simulink model "openWaterModel"  (R2020a)
settings: Solver=FixedStepAuto  StartTime=0.0  StopTime=inf  FixedStep=Ts  RelTol=1e-3  EnableMultiTasking=on
values from neighbouring files (symbols this model uses):
  ctrlMap =     [init_Kite.mat]
  Ts = 0.01    [init_Kite.mat]
undefined symbols (not defined in the file or in its folder): initializeBussesFromBlock, IO397, standard
libraries: xpcutilitieslib x172, hdlsllib x100, simulink x36, dspsigops x13, slrtlib x4, xpcseriallib x3, speedgoatlib_fpga_analog_io x2, xpcrtudplib x2, speedgoatlib_fpga_dio x1, speedgoatlib_fpga_quadrature x1, speedgoatlib_IO581 x1, speedgoatlib_fpga x1
(part 2 of 4)

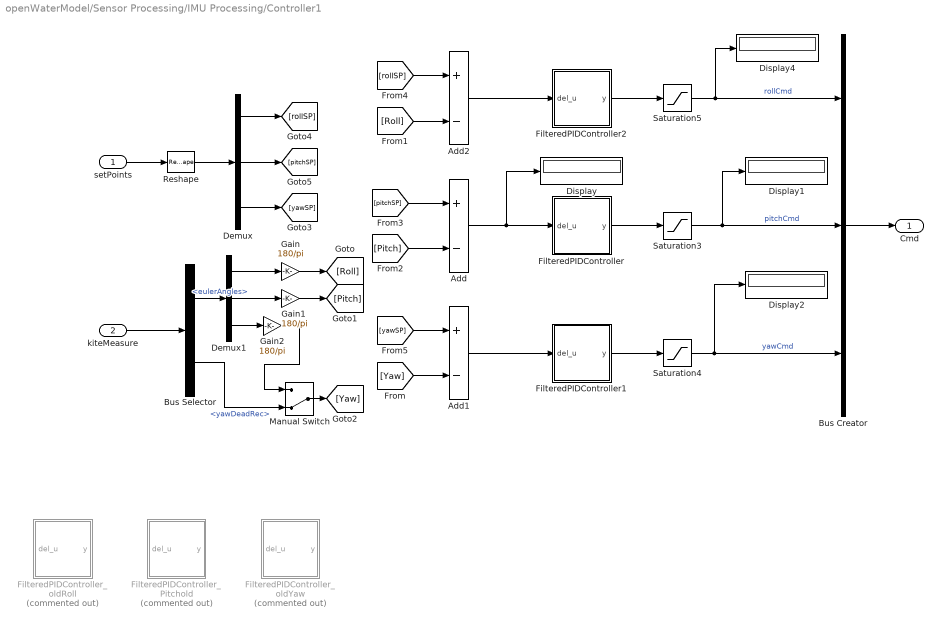
== system openWaterModel/Sensor Processing/IMU Processing/Controller1 ==
  setPoints : Inport
  kiteMeasure : Inport  Port=2
  Add : Sum  Inputs=+-
  Add1 : Sum  Inputs=+-
  Add2 : Sum  Inputs=+-
  Bus Creator : BusCreator  Inputs=3
  Bus Selector : BusSelector  OutputSignals=eulerAngles,yawDeadRec
  Demux : Demux  Outputs=3
  Demux1 : Demux  Outputs=3
  Display{,1..2,4} (4 alike) : Display
  FilteredPIDController : Subsystem  mask{Kp=1, Kd=0, tau=1, Ki=0}
      mask prompts: Kp "Proportional Gain"; Kd "Derivative Gain"; tau "Time constant"; Ki "Integral Gain"
  FilteredPIDController1 : Subsystem  mask{Kp=1, Kd=0, tau=1, Ki=0}
      mask prompts: Kp "Proportional Gain"; Kd "Derivative Gain"; tau "Time constant"; Ki "Integral Gain"
  FilteredPIDController2 : Subsystem  mask{Kp=1, Kd=0, tau=1, Ki=0}
      mask prompts: Kp "Proportional Gain"; Kd "Derivative Gain"; tau "Time constant"; Ki "Integral Gain"
  FilteredPIDController_Pitchold : Subsystem  Commented=on  mask{Kp=1, Kd=0, tau=1, Ki=0}
      mask prompts: Kp "Proportional Gain"; Kd "Derivative Gain"; tau "Time constant"; Ki "Integral Gain"
  FilteredPIDController_oldRoll : Subsystem  Commented=on  mask{Kp=1, Kd=0, tau=1, Ki=0}
      mask prompts: Kp "Proportional Gain"; Kd "Derivative Gain"; tau "Time constant"; Ki "Integral Gain"
  FilteredPIDController_oldYaw : Subsystem  Commented=on  mask{Kp=1, Kd=0, tau=1, Ki=0}
      mask prompts: Kp "Proportional Gain"; Kd "Derivative Gain"; tau "Time constant"; Ki "Integral Gain"
  Gain : Gain  Gain=180/pi
  Gain1 : Gain  Gain=180/pi
  Gain2 : Gain  Gain=180/pi
  Manual Switch : ManualSwitch  CurrentSetting=0
  Reshape : Reshape  OutputDimensionality=Column vector (2-D)
  Saturation3 : Saturate  UpperLimit=30  LowerLimit=-30
  Saturation4 : Saturate  UpperLimit=29  LowerLimit=-29
  Saturation5 : Saturate  UpperLimit=30  LowerLimit=-30
  Cmd : Outport
  wires:
  [Pitch] -> Add/2
  [Yaw] -> Add1/2
  [yawSP] -> Add1/1
  Demux/3 -> [yawSP]
  [pitchSP] -> Add/1
  kiteMeasure/1 -> Bus Selector/1
  Saturation4/1 -> Display2/1, Bus Creator/3  "yawCmd"
  Saturation5/1 -> Display4/1, Bus Creator/1  "rollCmd"
  Bus Creator/1 -> Cmd/1
  Reshape/1 -> Demux/1
  setPoints/1 -> Reshape/1
  Add/1 -> FilteredPIDController/1(del_u), Display/1
  [rollSP] -> Add2/1
  [Roll] -> Add2/2
  Demux/2 -> [pitchSP]
  Demux/1 -> [rollSP]
  Bus Selector/1 -> Demux1/1  "<eulerAngles>"
  Demux1/1 -> Gain/1
  Demux1/2 -> Gain1/1
  Demux1/3 -> Gain2/1
  Saturation3/1 -> Display1/1, Bus Creator/2  "pitchCmd"
  FilteredPIDController/1(y) -> Saturation3/1
  FilteredPIDController2/1(y) -> Saturation5/1
  Add2/1 -> FilteredPIDController2/1(del_u)
  FilteredPIDController1/1(y) -> Saturation4/1
  Add1/1 -> FilteredPIDController1/1(del_u)
  Gain/1 -> [Roll]
  Gain1/1 -> [Pitch]
  Bus Selector/2 -> Manual Switch/2  "<yawDeadRec>"
  Gain2/1 -> Manual Switch/1
  Manual Switch/1 -> [Yaw]

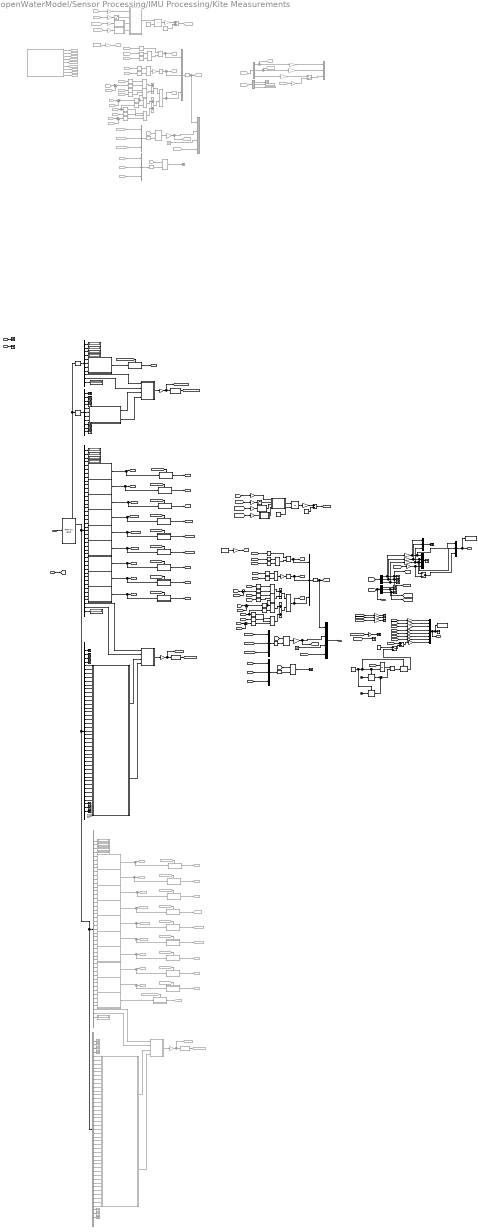
== system openWaterModel/Sensor Processing/IMU Processing/Kite Measurements  ==
  note: Dead Reconing Yaw
  note: Tranformation from IMU euler angles w.r.t NED to Body euler angles w.r.t Ground. Transformation from acc / angular rate in the IMU to acc / angular rate in the Body.
  note: Debug
  note: Tranformation from IMU euler angles w.r.t NED to Body euler angles w.r.t Ground. Transformation from acc / angular rate in the IMU to acc / angular rate in the Body.
  note: Serial Data Recieve
  serialData : Inport
  DcM : Inport  Port=2
  gndStnEul : Inport  Port=3
  winchCmd : Inport  Port=4
  Add : Sum  Commented=on
  Add1 : Sum  Commented=on
  Add2 : Sum  Commented=on  Inputs=+-
  Add3 : Sum
  Add4 : Sum
  Add5 : Sum  Inputs=+-
  Add6 : Sum  Inputs=+-
  Bus Creator1 : BusCreator  Commented=on  Inputs=4
  Bus Creator2 : BusCreator  Inputs=4
  Cast To Boolean : DataTypeConversion  OutDataTypeStr=boolean
  Cast To Boolean1 : DataTypeConversion  OutDataTypeStr=boolean
  Cast To Boolean2 : DataTypeConversion  Commented=on  OutDataTypeStr=boolean
  Clock : Clock
  Clock1 : Clock
  Constant : Constant  Value=0
  Cos{1..2,4,6,10..11} (6 alike) : Trigonometry  Commented=on
  Cos{3,5,7..9,12..13} (7 alike) : Trigonometry  Commented=on  Operator=cos
  Cos{14..16,19,21,23} (6 alike) : Trigonometry
  Cos{17..18,20,22,24..26} (7 alike) : Trigonometry  Operator=cos
  Demux : Demux  Outputs=43
  Demux1 : Demux  Commented=on  Outputs=3
  Demux2 : Demux  Commented=on  Outputs=3
  Demux3 : Demux  Outputs=3
  Demux4 : Demux  Outputs=3
  Demux5 : Demux  Outputs=43
  Demux6 : Demux  Outputs=11
  Demux7 : Demux  Outputs=11
  Demux8 : Demux  Commented=on  Outputs=47
  Demux9 : Demux  Commented=on  Outputs=47
  Display{,1..9} (10 alike) : Display
      Display settings: Format=hex (Stored Integer)
      Display2 settings: Format=hex (Stored Integer)
      Display3 settings: Format=hex (Stored Integer)
      Display4 settings: Format=hex (Stored Integer)
      Display5 settings: Format=hex (Stored Integer)
      Display6 settings: Format=hex (Stored Integer)
      Display7 settings: Format=hex (Stored Integer)
      Display8 settings: Format=hex (Stored Integer)
  Display{10..14} (5 alike) : Display  Commented=on
      Display10 settings: Format=hex (Stored Integer)
      Display12 settings: Format=hex (Stored Integer)
      Display13 settings: Format=hex (Stored Integer)
      Display14 settings: Format=hex (Stored Integer)
  Divide : Product  Inputs=*/
  Enabled Subsystem : Subsystem  TreatAsAtomicUnit=on
  Enabled Subsystem1 : Subsystem  TreatAsAtomicUnit=on
  Enabled Subsystem10 : Subsystem  Commented=on  TreatAsAtomicUnit=on
  Enabled Subsystem11 : Subsystem  Commented=on  TreatAsAtomicUnit=on
  Enabled Subsystem12 : Subsystem  Commented=on  TreatAsAtomicUnit=on
  Enabled Subsystem13 : Subsystem  Commented=on  TreatAsAtomicUnit=on
  Enabled Subsystem14 : Subsystem  Commented=on  TreatAsAtomicUnit=on
  Enabled Subsystem15 : Subsystem  Commented=on  TreatAsAtomicUnit=on
  Enabled Subsystem16 : Subsystem  Commented=on  TreatAsAtomicUnit=on
  Enabled Subsystem17 : Subsystem  Commented=on  TreatAsAtomicUnit=on
  Enabled Subsystem18 : Subsystem  Commented=on  TreatAsAtomicUnit=on
  Enabled Subsystem19 : Subsystem  Commented=on  TreatAsAtomicUnit=on
  Enabled Subsystem2 : Subsystem  TreatAsAtomicUnit=on
  Enabled Subsystem3 : Subsystem  TreatAsAtomicUnit=on
  Enabled Subsystem4 : Subsystem  TreatAsAtomicUnit=on
  Enabled Subsystem5 : Subsystem  TreatAsAtomicUnit=on
  Enabled Subsystem6 : Subsystem  TreatAsAtomicUnit=on
  Enabled Subsystem7 : Subsystem  TreatAsAtomicUnit=on
  Enabled Subsystem8 : Subsystem  TreatAsAtomicUnit=on
  Enabled Subsystem9 : Subsystem  TreatAsAtomicUnit=on
  "FIFO bin read " : xpcseriallib/FIFO bin read   header={[0x47 0xBB 0x3C 0x2B] [0x58 0xCC 0x4D 0x3C]}  lengths=[42 10]  hold=Hold last output if no new data  enable=off  maxsize=42  outputtype=8 bit uint null terminated  sampletime=0.01
      settings: SourceProductBaseCode=XP
  Fletcher16 Checksum : Subsystem
  Fletcher16 Checksum1 : Subsystem
  Fletcher16 Checksum2 : Subsystem  Commented=on
  From1 : From  Commented=on  GotoTag=yawDeadRec
  From10 : From  Commented=on  GotoTag=DcM
  From2 : From  Commented=on  GotoTag=eulVector
  From3 : From  Commented=on  GotoTag=rateVector
  From35 : From  Commented=on  GotoTag=psiG
  From{36,40,42..43,53} (5 alike) : From  Commented=on  GotoTag=thetaIMU
  From37 : From  Commented=on  GotoTag=DcM
  From38 : From  Commented=on  GotoTag=pIMU
  From{39,41,44,54..55} (5 alike) : From  Commented=on  GotoTag=phiIMU
  From4 : From  Commented=on  GotoTag=roll
  From{45,59..60,72,87,89..91,97} (9 alike) : From  Commented=on  GotoTag=checksumEnable
  From46 : From  Commented=on  GotoTag=rIMU
  From47 : From  Commented=on  GotoTag=axIMU
  From48 : From  Commented=on  GotoTag=ayIMU
  From49 : From  Commented=on  GotoTag=azIMU
  From5 : From  Commented=on  GotoTag=pitch
  From50 : From  Commented=on  GotoTag=psiG
  From51 : From  Commented=on  GotoTag=psiIMU
  From52 : From  Commented=on  GotoTag=psiIMU
  From56 : From  Commented=on  GotoTag=psiG
  From57 : From  Commented=on  GotoTag=psiIMU
  From58 : From  Commented=on  GotoTag=qIMU
  From6 : From  Commented=on  GotoTag=q
  From7 : From  Commented=on  GotoTag=r
  From8 : From  Commented=on  GotoTag=yawDeadRec
  From92 : From  Commented=on  GotoTag=checksumEnablePressure
  Gain : Gain  Commented=on  Gain=-1
  Gain1 : Gain  Gain=-1
  Gain{10,15,21..23} (5 alike) : Gain  Commented=on  Gain=180/pi
  Gain{4,11..14,25..27,32..33} (10 alike) : Gain  Gain=180/pi
  Gain16 : Gain  Commented=on
  Gain{3,5,17..19,24,29..30} (8 alike) : Gain
  Gain2 : Gain  Commented=on  Gain=-1
  Gain20 : Gain  Gain=-1
  Gain28 : Gain  Gain=1.01972
  Gain31 : Gain  Commented=on
  Gain{34..37} (4 alike) : Gain  Gain=pi/180
  Gain{6..9} (4 alike) : Gain  Commented=on  Gain=pi/180
  Goto18 : Goto  Commented=on  GotoTag=phiIMU
  Goto19 : Goto  Commented=on  GotoTag=psiIMU
  Goto20 : Goto  Commented=on  GotoTag=pIMU
  Goto22 : Goto  Commented=on  GotoTag=qIMU
  Goto23 : Goto  Commented=on  GotoTag=rIMU
  Goto24 : Goto  Commented=on  GotoTag=axIMU
  Goto25 : Goto  Commented=on  GotoTag=ayIMU
  Goto26 : Goto  Commented=on  GotoTag=azIMU
  Goto27 : Goto  Commented=on  GotoTag=thetaIMU
  Goto28 : Goto  Commented=on  GotoTag=psiG
  Goto29 : Goto  Commented=on  GotoTag=phi
  Goto3 : Goto  Commented=on  GotoTag=roll
  Goto30 : Goto  Commented=on  GotoTag=theta
  Goto31 : Goto  Commented=on  GotoTag=psi
  Goto32 : Goto  Commented=on  GotoTag=eulVector
  Goto33 : Goto  Commented=on  GotoTag=rateVector
  Goto4 : Goto  Commented=on  GotoTag=pitch
  Goto49 : Goto  Commented=on  GotoTag=thetaRaw
  Goto5 : Goto  Commented=on  GotoTag=q
  Goto50 : Goto  Commented=on  GotoTag=psiRaw
  Goto51 : Goto  Commented=on  GotoTag=pRaw
  Goto52 : Goto  Commented=on  GotoTag=qRaw
  Goto53 : Goto  Commented=on  GotoTag=rRaw
  Goto55 : Goto  Commented=on  GotoTag=ayRaw
  Goto56 : Goto  Commented=on  GotoTag=azRaw
  Goto57 : Goto  Commented=on  GotoTag=checksumEnable
  Goto58 : Goto  Commented=on  GotoTag=phiIMU
  Goto59 : Goto  Commented=on  GotoTag=psiIMU
  Goto6 : Goto  Commented=on  GotoTag=r
  Goto60 : Goto  Commented=on  GotoTag=pIMU
  Goto61 : Goto  Commented=on  GotoTag=CSisMatch
  Goto62 : Goto  Commented=on  GotoTag=qIMU
  Goto63 : Goto  Commented=on  GotoTag=rIMU
  Goto64 : Goto  Commented=on  GotoTag=axIMU
  Goto66 : Goto  Commented=on  GotoTag=ayIMU
  Goto67 : Goto  Commented=on  GotoTag=azIMU
  Goto68 : Goto  Commented=on  GotoTag=thetaIMU
  Goto69 : Goto  Commented=on  GotoTag=axRaw
  Goto7 : Goto  Commented=on  GotoTag=yawDeadRec
  Goto70 : Goto  Commented=on  GotoTag=phiRaw
  Goto71 : Goto  Commented=on  GotoTag=pres
  Ground : Ground  Commented=on
  Ground1 : Ground
  Ground2 : Ground  Commented=on
  Integrator : Integrator  Commented=on  ExternalReset=either
  Integrator1 : Integrator  ExternalReset=either
  Integrator2 : Integrator  ExternalReset=either
  MATLAB Function : MATLAB Function  Commented=on  TreatAsAtomicUnit=on
  MATLAB Function1 : MATLAB Function  Commented=on  TreatAsAtomicUnit=on
  MATLAB Function2 : MATLAB Function  Commented=on  TreatAsAtomicUnit=on
  MATLAB Function3 : MATLAB Function  TreatAsAtomicUnit=on
  MATLAB Function4 : MATLAB Function  TreatAsAtomicUnit=on
  MATLAB Function5 : MATLAB Function  TreatAsAtomicUnit=on
  MATLAB Function6 : MATLAB Function  TreatAsAtomicUnit=on
  MATLAB Function7 : MATLAB Function  TreatAsAtomicUnit=on
  MATLAB Function8 : MATLAB Function  Commented=on  TreatAsAtomicUnit=on
  Manual Switch : ManualSwitch  Commented=on  CurrentSetting=0
  Manual Switch1 : ManualSwitch  CurrentSetting=0
  Manual Switch2 : ManualSwitch
  Matrix Multiply1 : Product  Multiplication=Matrix(*)
  Matrix Multiply2 : Product  Commented=on  Multiplication=Matrix(*)
  Matrix Multiply3 : Product  Commented=on  Multiplication=Matrix(*)
  Matrix Multiply4 : Product  Multiplication=Matrix(*)
  Mux{,5..7} (4 alike) : Mux  Commented=on  Inputs=3
  Mux{1,4,8..10} (5 alike) : Mux  Inputs=3
  Mux2 : Mux
  Mux3 : Mux  Inputs=8
  PoolToNorthAngle : Constant  Commented=on  Value=2.4070
  PoolToNorthAngle1 : Constant  Value=2.4070
  Product{1..2,5..6} (4 alike) : Product  Commented=on
  Product10 : Product  Inputs=3
  Product{7..8,11..12} (4 alike) : Product
  Product3 : Product  Commented=on  Inputs=3
  Product4 : Product  Commented=on  Inputs=3
  Product9 : Product  Inputs=3
  Reshape1 : Reshape  OutputDimensionality=Column vector (2-D)
  Reshape2 : Reshape  Commented=on  OutputDimensionality=Column vector (2-D)
  Reshape3 : Reshape  Commented=on  OutputDimensionality=Column vector (2-D)
  Reshape4 : Reshape  Commented=on  OutputDimensionality=Column vector (2-D)
  Reshape5 : Reshape  OutputDimensionality=Column vector (2-D)
  Reshape6 : Reshape  OutputDimensionality=Column vector (2-D)
  Sample and Hold : dspsigops/Sample and Hold  trig=Rising edge  initCond=0  latchinput=off
  Sample and Hold1 : dspsigops/Sample and Hold  trig=Falling edge  initCond=999999  latchinput=off
  Sample and Hold2 : dspsigops/Sample and Hold  trig=Falling edge  initCond=0  latchinput=off
  Saturation : Saturate  Commented=on  UpperLimit=pi/2-0.1  LowerLimit=-pi/2+0.1
  Saturation1 : Saturate  UpperLimit=pi/2-0.1  LowerLimit=-pi/2+0.1
  Scope 1 : slrtlib/Displays and Logging/Scope   scopeno=3  scopetype=Target  autostart=on  viewmode=Numerical  formatstr='%15.6f'  grid=on  ylimits=[-100,100]  nosamples=scopeSamples  noprepostsamples=0  interleave=scopeDecimaton  triggermode=FreeRun  triggersignal=1  trigsignalfromport=off  triggerlevel=0.0  triggerslope=Either  triggerscope=1  triggersample=0  filename=data.dat  mode=Lazy  writesize=512  autorestart=off  dynamicfilemode=off  maxwritefilesize=512*1024^2
  Scope 2 : slrtlib/Displays and Logging/Scope   scopeno=1  scopetype=Target  autostart=on  viewmode=Graphical sliding  formatstr='%15.6f'  grid=on  ylimits=[-100,100]  nosamples=scopeSamples  noprepostsamples=0  interleave=scopeDecimaton  triggermode=FreeRun  triggersignal=1  trigsignalfromport=off  triggerlevel=0.0  triggerslope=Either  triggerscope=1  triggersample=0  filename=data.dat  mode=Lazy  writesize=512  autorestart=off  dynamicfilemode=off  maxwritefilesize=512*1024^2
  Selector : Selector  InputPortWidth=43  IndexOptions=Index vector (dialog)  Indices=[1 2 3 4 5 6 7 8 9 10 11]  OutputSizes=1
  Selector1 : Selector  InputPortWidth=43  IndexOptions=Index vector (dialog)  Indices=[1 2 3 4 5 6 7 8 9 10 11]  OutputSizes=1
  Serial Data Recieve : Subsystem  Commented=on
  Sin1 : Trigonometry
  Sin4 : Trigonometry  Commented=on
  Sum : Sum  Inputs=|-+
  Sum1 : Sum  Commented=on  Inputs=|+-
  Sum2 : Sum  Commented=on  Inputs=|+-
  Sum3 : Sum  Commented=on  Inputs=|+-
  Sum4 : Sum  Inputs=|+-
  Sum5 : Sum  Inputs=|+-
  Sum6 : Sum  Inputs=|+-
  Terminator{,1..3,5..6,8..22,27..29,33..39} (31 alike) : Terminator
  Terminator{4,7,23..26,30..32} (9 alike) : Terminator  Commented=on
  Trigonometric Function : Trigonometry  Commented=on  Operator=atan2
  Trigonometric Function1 : Trigonometry  Commented=on  Operator=asin
  Trigonometric Function2 : Trigonometry  Commented=on  Operator=atan2
  Trigonometric Function3 : Trigonometry  Operator=atan2
  Trigonometric Function4 : Trigonometry  Operator=asin
  Trigonometric Function5 : Trigonometry  Operator=atan2
  airPressure : Constant  Value=1022
  binary2double : Subsystem
  binary2double1 : Subsystem
  binary2double10 : Subsystem  Commented=on
  binary2double11 : Subsystem  Commented=on
  binary2double12 : Subsystem  Commented=on
  binary2double13 : Subsystem  Commented=on
  binary2double14 : Subsystem  Commented=on
  binary2double15 : Subsystem  Commented=on
  binary2double16 : Subsystem  Commented=on
  binary2double17 : Subsystem  Commented=on
  binary2double18 : Subsystem  Commented=on
  binary2double19 : Subsystem  Commented=on
  binary2double2 : Subsystem
  binary2double3 : Subsystem
  binary2double4 : Subsystem
  binary2double5 : Subsystem
  binary2double6 : Subsystem
  binary2double7 : Subsystem
  binary2double8 : Subsystem
  binary2double9 : Subsystem
  eulRates : Gain  Gain=180/pi
  yawBias : Constant  Commented=on  Value=0
  yawBias1 : Constant  Value=0
  yawEstimateTrigger : Constant  Commented=on  Value=0
  yawEstimateTrigger1 : Constant
  kiteMeasure : Outport
  eul : Outport  Port=2
  angVel : Outport  Port=3
  MC_rawData : Outport  Port=4
  wires:
  From2/1 -> Demux1/1
  From3/1 -> Demux2/1
  Demux1/3 -> Gain23/1
  Demux1/1 -> Gain21/1, Goto3/1
  Demux2/3 -> Goto6/1  "r"
  Demux2/2 -> Goto5/1  "q"
  Demux2/1 -> Terminator4/1  "p"
  Gain9/1 -> MATLAB Function1/1(u)  "kiteYawRate_rad"
  Gain8/1 -> MATLAB Function2/1(u)  "kitePitchRate_rad"
  From6/1 -> Gain8/1
  From5/1 -> Gain7/1
  Saturation/1 -> MATLAB Function/2(theta)  "kitePitch_rad"
  Gain6/1 -> MATLAB Function/1(phi)  "kiteRoll_rad"
  Integrator/1 -> Gain10/1
  From7/1 -> Gain9/1
  From4/1 -> Gain6/1
  Gain7/1 -> Saturation/1
  yawEstimateTrigger/1 -> Integrator/2
  MATLAB Function/1(psi_dot) -> Integrator/1
  yawBias/1 -> Add/2
  Add/1 -> Goto7/1
  Gain10/1 -> Add/1  "rollRaw"
  MATLAB Function1/1(y) -> MATLAB Function/4(r)
  MATLAB Function2/1(y) -> MATLAB Function/3(q)
  Gain21/1 -> Mux/1  "rollDeg"
  Gain22/1 -> Mux/2  "pitchDeg"
  Gain23/1 -> Manual Switch/1  "yawIMU"
  Gain16/1 -> Manual Switch/2  "yawDeadRec"
  PoolToNorthAngle/1 -> Gain2/1
  Trigonometric Function/1 -> Mux5/1, Goto29/1
  Product2/1 -> Gain/1
  Cos2/1 -> Product2/1
  Cos3/1 -> Product2/2
  From42/1 -> Cos3/1
  From41/1 -> Cos2/1
  Trigonometric Function1/1 -> Mux5/2, Goto30/1
  Add2/1 -> Trigonometric Function2/1
  Sin4/1 -> Product4/1
  From44/1 -> Cos7/1, Sin4/1
  Mux5/1 -> Reshape2/1
  Trigonometric Function2/1 -> Goto31/1, Mux5/3
  Gain15/1 -> Goto33/1, Bus Creator1/2  "gyroRates"
  From58/1 -> Mux6/2
  Ground2/1 -> Bus Creator1/3  "Pressure (Pa)"
  From37/1 -> Matrix Multiply2/1
  Reshape3/1 -> Matrix Multiply2/2
  Reshape2/1 -> Bus Creator1/1, Goto32/1  "eulerAngles"
  Mux6/1 -> Reshape3/1
  Matrix Multiply2/1 -> Gain15/1
  From46/1 -> Mux6/3
  From38/1 -> Mux6/1
  From47/1 -> Mux7/1
  From49/1 -> Mux7/3
  Mux7/1 -> Reshape4/1
  Reshape4/1 -> Matrix Multiply3/2
  From10/1 -> Matrix Multiply3/1
  From48/1 -> Mux7/2
  Matrix Multiply3/1 -> Terminator7/1  "accBody"
  Gain/1 -> Trigonometric Function1/1
  Product1/1 -> Trigonometric Function/2
  Cos1/1 -> Trigonometric Function/1
  From36/1 -> Cos1/1
  From39/1 -> Cos8/1
  From40/1 -> Cos9/1
  Cos9/1 -> Product1/2
  Cos8/1 -> Product1/1
  From50/1 -> Sum1/1
  From51/1 -> Sum1/2
  Sum1/1 -> Cos5/1
  Cos5/1 -> Product4/3
  From43/1 -> Cos6/1
  Cos6/1 -> Product4/2
  Product4/1 -> Add1/2
  Product5/1 -> Add1/1
  Cos7/1 -> Product5/2
  Cos10/1 -> Product3/3, Product5/1
  From52/1 -> Sum2/2
  From35/1 -> Sum2/1
  Sum2/1 -> Cos10/1
  Add1/1 -> Trigonometric Function2/2
  From53/1 -> Cos4/1
  From54/1 -> Cos11/1
  Cos11/1 -> Product3/2
  Cos4/1 -> Product3/1
  Product3/1 -> Add2/2
  From55/1 -> Cos12/1
  From56/1 -> Sum3/1
  From57/1 -> Sum3/2
  Sum3/1 -> Cos13/1
  Product6/1 -> Add2/1
  Cos13/1 -> Product6/2
  Cos12/1 -> Product6/1
  Gain2/1 -> Goto28/1
  From8/1 -> Gain16/1
  From1/1 -> Bus Creator1/4  "yawDeadRec"
  Manual Switch/1 -> Mux/3  "yawDeg"
  Demux1/2 -> Goto4/1, Gain22/1
  Serial Data Recieve/1(rawRollChecked) -> Goto18/1
  Serial Data Recieve/2(rawPitchChecked) -> Goto27/1
  Serial Data Recieve/3(rawRollChecked1) -> Goto19/1
  Serial Data Recieve/4(rawPchecked) -> Goto20/1
  Serial Data Recieve/5(rawQchecked) -> Goto22/1
  Serial Data Recieve/6(rawRchecked) -> Goto23/1
  Serial Data Recieve/7(rawAxChecked) -> Goto24/1
  Serial Data Recieve/8(rawAyChecked) -> Goto25/1
  Serial Data Recieve/9(rawAzChecked) -> Goto26/1
  gndStnEul/1 -> Terminator/1
  winchCmd/1 -> Terminator1/1
  airPressure/1 -> Manual Switch2/1
  Enabled Subsystem10/1(Out1) -> Goto58/1  "rawRollChecked"
  Demux6/4 -> Display5/1
  Gain12/1 -> Terminator29/1  "p"
  Demux9/24 -> Fletcher16 Checksum2/20(In20)
  Demux4/3 -> [kiteR], Terminator36/1  "kiteR"
  Demux/7 -> binary2double/3(In3)
  Gain34/1 -> MATLAB Function3/1(phi)  "kiteRoll_rad"
  [yawDeadRec] -> Bus Creator2/4  "yawDeadRec"
  Demux8/16 -> binary2double12/4(In4)
  Demux8/37 -> binary2double18/1(In1)
  [thetaIMU] -> Cos14/1
  Demux9/13 -> Fletcher16 Checksum2/9(In9)
  Demux9/39 -> Fletcher16 Checksum2/35(In35)
  Cos23/1 -> Product10/2
  Demux8/27 -> binary2double15/3(In3)
  Demux9/42 -> Fletcher16 Checksum2/38(In38)
  Add4/1 -> Trigonometric Function5/2
  Cast To Boolean2/1 -> Goto57/1
  Demux8/4 -> Display10/1
  binary2double16/1(Double) -> Enabled Subsystem16/1(Double), Goto69/1  "rawAx"
  Demux5/25 -> Fletcher16 Checksum/21(In21)
  Mux4/1 -> Terminator38/1
  [DcM] -> Matrix Multiply1/1
  Gain31/1 -> Goto61/1, Cast To Boolean2/1  "checksumIsMatch"
  Reshape1/1 -> Bus Creator2/1, [eulVector]  "eulerAngles"
  From91/1 -> Enabled Subsystem18/Enable
  Demux5/14 -> Fletcher16 Checksum/10(In10)
  Demux/11 -> binary2double1/3(In3)
  Add6/1 -> Gain28/1
  Demux3/2 -> [kitePitch], Terminator5/1, Gain26/1  "kitePitch"
  Gain11/1 -> Mux3/1  "phi"
  Demux/41 -> MATLAB Function6/1(cSumInB1)  "cSumInB1"
  Demux/28 -> binary2double5/4(In4)
  Demux8/24 -> binary2double14/4(In4)
  Mux2/1 -> Terminator15/1
  Demux7/1 -> Terminator3/1
  Enabled Subsystem1/1(Out1) -> [thetaIMU]  "rawPitchChecked"
  [thetaIMU] -> Cos26/1
  Demux6/10 -> MATLAB Function7/2(cSumInB2)
  Gain37/1 -> MATLAB Function4/1(u)  "kiteYawRate_rad"
  [pRaw] -> Gain12/1  "pRaw"
  [checksumEnable] -> Enabled Subsystem3/Enable
  [checksumEnable] -> Enabled Subsystem6/Enable
  [ayIMU] -> Mux10/2
  binary2double3/1(Double) -> Enabled Subsystem3/1(Double), [pRaw]  "rawP"
  [checksumEnable] -> Enabled Subsystem8/Enable
  Gain24/1 -> [CSisMatch], Cast To Boolean/1  "checksumIsMatch"
  Demux8/43 -> binary2double19/3(In3)
  [rIMU] -> Mux9/3
  From59/1 -> Enabled Subsystem12/Enable
  Matrix Multiply1/1 -> eulRates/1
  Gain33/1 -> Mux3/3  "psi"
  MATLAB Function3/1(psi_dot) -> Integrator1/1
  [pres] -> Gain17/1
  Mux9/1 -> Reshape5/1
  [pIMU] -> Mux9/1
  [phiIMU] -> Cos19/1
  Trigonometric Function3/1 -> Mux8/1, [phi]
  Demux9/9 -> Fletcher16 Checksum2/5(In5)
  Demux9/11 -> Fletcher16 Checksum2/7(In7)
  [rRaw] -> Gain14/1  "rRaw"
  MATLAB Function6/1(checksumIsMatching) -> Gain24/1
  Mux8/1 -> Reshape1/1
  Demux8/5 -> binary2double10/1(In1)
  Demux8/19 -> binary2double13/3(In3)
  [ayRaw] -> Gain18/1
  Demux5/6 -> Fletcher16 Checksum/2(In2)
  Cast To Boolean/1 -> [checksumEnable]
  [psiG] -> Sum4/1
  Manual Switch1/1 -> Mux1/3  "yawChosen"
  From87/1 -> Enabled Subsystem15/Enable
  MATLAB Function4/1(y) -> MATLAB Function3/4(r)
  binary2double9/1(Double) -> Enabled Subsystem9/1(Double)  "rawPressure"
  Demux/40 -> binary2double8/4(In4)
  [checksumEnablePressure] -> Enabled Subsystem9/Enable
  [kiteRoll] -> Gain34/1
  Demux/15 -> binary2double2/3(In3)
  Cos17/1 -> Product12/1
  binary2double7/1(Double) -> Enabled Subsystem7/1(Double), [ayRaw]  "rawAy"
  [yawDeadRec] -> Gain5/1
  [thetaIMU] -> Cos23/1
  Demux/38 -> binary2double8/2(In2)
  Enabled Subsystem9/1(Out1) -> [pres]  "rawAzChecked"
  Demux8/9 -> binary2double11/1(In1)
  Product8/1 -> Gain1/1
  Gain28/1 -> Mux3/8  "depth_cm"
  From97/1 -> Enabled Subsystem10/Enable
  Gain26/1 -> Mux4/2, Mux1/2, Mux2/2  "pitch"
  Gain29/1 -> Terminator27/1  "CSIsMatchPress"
  Demux5/27 -> Fletcher16 Checksum/23(In23)
  Gain5/1 -> Mux2/4, Manual Switch1/2  "yawDeadRec"
  Demux5/20 -> Fletcher16 Checksum/16(In16)
  [axIMU] -> Mux10/1
  [checksumEnable] -> Enabled Subsystem2/Enable
  Demux8/26 -> binary2double15/2(In2)
  Demux5/1 -> Terminator11/1
  Demux8/34 -> binary2double17/2(In2)
  Mux3/1 -> MC_rawData/1, Scope 1/1, Terminator35/1
  Sample and Hold1/1 -> Sum/2
  Enabled Subsystem15/1(Out1) -> Goto63/1  "rawRchecked"
  [qRaw] -> Gain13/1  "qRaw"
  [qIMU] -> Mux9/2
  Sum/1 -> Divide/2
  Demux5/16 -> Fletcher16 Checksum/12(In12)
  Fletcher16 Checksum1/2(Out2) -> MATLAB Function7/4(cSumCalcB2)  "cSumCalcB2"
  [azRaw] -> Gain19/1
  Demux8/31 -> binary2double16/3(In3)
  Demux5/40 -> Fletcher16 Checksum/36(In36)
  [checksumEnable] -> Enabled Subsystem4/Enable
  Demux9/37 -> Fletcher16 Checksum2/33(In33)
  Demux/5 -> binary2double/1(In1)
  Demux5/15 -> Fletcher16 Checksum/11(In11)
  [CSisMatchPressure] -> Gain29/1
  Demux6/1 -> Display8/1
  "FIFO bin read "/2 -> Selector1/1, Selector/1
  Gain35/1 -> Saturation1/1
  Demux9/12 -> Fletcher16 Checksum2/8(In8)
  [thetaIMU] -> Cos20/1
  Fletcher16 Checksum/1(Out1) -> MATLAB Function6/3(cSumCalcB1)  "cSumCalcB1"
  Sample and Hold2/1 -> Manual Switch2/2  "pCalib"
  Demux8/46 -> MATLAB Function8/2(cSumInB2)  "cSumInB2"
  Demux6/9 -> MATLAB Function7/1(cSumInB1)
  Demux8/6 -> binary2double10/2(In2)
  Enabled Subsystem7/1(Out1) -> [ayIMU]  "rawAyChecked"
  Gain32/1 -> Mux3/2  "theta"
  Enabled Subsystem13/1(Out1) -> Goto60/1  "rawPchecked"
  Demux/34 -> binary2double7/2(In2)
  Demux/37 -> binary2double8/1(In1)
  Demux5/5 -> Fletcher16 Checksum/1(In1)
  Gain20/1 -> [psiG]
  Demux5/29 -> Fletcher16 Checksum/25(In25)
  binary2double/1(Double) -> Enabled Subsystem/1(Double), [phiRaw]  "rawRoll"
  Trigonometric Function4/1 -> Mux8/2, [theta]
  Cos15/1 -> Product9/3, Product11/1
  Integrator1/1 -> Gain4/1
  binary2double17/1(Double) -> Enabled Subsystem17/1(Double), Goto55/1  "rawAy"
  Demux3/1 -> Gain25/1, [kiteRoll], Terminator2/1  "kiteRoll"
  Demux9/18 -> Fletcher16 Checksum2/14(In14)
  Demux/27 -> binary2double5/3(In3)
  [kitePitch] -> Gain35/1
  Demux9/23 -> Fletcher16 Checksum2/19(In19)
  Demux3/3 -> Gain27/1, Terminator6/1  "kiteYaw"
  Demux8/42 -> binary2double19/2(In2)
  Enabled Subsystem2/1(Out1) -> [psiIMU]  "rawRollChecked"
  [axRaw] -> Gain30/1
  Demux5/43 -> Terminator18/1
  Trigonometric Function5/1 -> [psi], Mux8/3
  Demux/35 -> binary2double7/3(In3)
  Demux9/32 -> Fletcher16 Checksum2/28(In28)
  Demux8/7 -> binary2double10/3(In3)
  Demux/25 -> binary2double5/1(In1)
  Demux/3 -> Display2/1
  [phiIMU] -> Cos17/1
  Gain36/1 -> MATLAB Function5/1(u)  "kitePitchRate_rad"
  Demux/26 -> binary2double5/2(In2)
  Demux/1 -> Display4/1
  binary2double8/1(Double) -> Enabled Subsystem8/1(Double), [azRaw]  "rawAz"
  Product7/1 -> Trigonometric Function3/2
  Demux/30 -> binary2double6/2(In2)
  Demux8/45 -> MATLAB Function8/1(cSumInB1)  "cSumInB1"
  Demux8/33 -> binary2double17/1(In1)
  Demux5/10 -> Fletcher16 Checksum/6(In6)
  Demux/12 -> binary2double1/4(In4)
  Demux8/12 -> binary2double11/4(In4)
  [eulVector] -> Demux3/1
  Demux5/13 -> Fletcher16 Checksum/9(In9)
  Demux5/12 -> Fletcher16 Checksum/8(In8)
  Demux5/24 -> Fletcher16 Checksum/20(In20)
  Demux5/23 -> Fletcher16 Checksum/19(In19)
  Demux8/36 -> binary2double17/4(In4)
  binary2double14/1(Double) -> Enabled Subsystem14/1(Double), Goto52/1  "rawQ"
  Demux5/35 -> Fletcher16 Checksum/31(In31)
  Demux5/39 -> Fletcher16 Checksum/35(In35)
  Demux7/4 -> Terminator19/1
  Product9/1 -> Add5/2
  Demux9/2 -> Terminator24/1
  Demux9/15 -> Fletcher16 Checksum2/11(In11)
  Demux/23 -> binary2double4/3(In3)
  binary2double13/1(Double) -> Enabled Subsystem13/1(Double), Goto51/1  "rawP"
  Demux9/44 -> Fletcher16 Checksum2/40(In40)
  Demux/32 -> binary2double6/4(In4)
  Demux/29 -> binary2double6/1(In1)
  [phiIMU] -> Cos16/1
  Demux5/38 -> Fletcher16 Checksum/34(In34)
  Demux8/29 -> binary2double16/1(In1)
  binary2double2/1(Double) -> Enabled Subsystem2/1(Double), [psiRaw]  "rawYaw"
  Reshape5/1 -> Matrix Multiply1/2
  Demux9/20 -> Fletcher16 Checksum2/16(In16)
  [pres] -> Add6/1
  [psiIMU] -> Sum5/2
  Enabled Subsystem19/1(Out1) -> Goto71/1  "pressure"
  Demux9/35 -> Fletcher16 Checksum2/31(In31)
  Manual Switch2/1 -> Add6/2
  Demux5/9 -> Fletcher16 Checksum/5(In5)
  Enabled Subsystem11/1(Out1) -> Goto68/1  "rawPitchChecked"
  [psiG] -> Sum5/1
  [azIMU] -> Mux10/3
  Gain19/1 -> Mux3/6  "az"
  [psiRaw] -> Gain33/1
  Demux/39 -> binary2double8/3(In3)
  Demux5/4 -> Terminator14/1
  [psiG] -> Sum6/1
  Demux7/7 -> Fletcher16 Checksum1/3(In3)
  Cos19/1 -> Product8/1
  Demux8/2 -> Display13/1
  Demux7/11 -> Terminator22/1
  Demux/16 -> binary2double2/4(In4)
  Gain14/1 -> Terminator34/1  "r"
  Cos26/1 -> Product7/2
  binary2double4/1(Double) -> Enabled Subsystem4/1(Double), [qRaw]  "rawQ"
  Demux9/36 -> Fletcher16 Checksum2/32(In32)
  Demux5/36 -> Fletcher16 Checksum/32(In32)
  Demux8/8 -> binary2double10/4(In4)
  Demux9/27 -> Fletcher16 Checksum2/23(In23)
  Fletcher16 Checksum/2(Out2) -> MATLAB Function6/4(cSumCalcB2)  "cSumCalcB2"
  Add3/1 -> [yawDeadRec]
  Demux9/21 -> Fletcher16 Checksum2/17(In17)
  Demux8/23 -> binary2double14/3(In3)
  [kiteR] -> Gain37/1
  Demux8/17 -> binary2double13/1(In1)
  Demux8/35 -> binary2double17/3(In3)
  Demux5/33 -> Fletcher16 Checksum/29(In29)
  Demux9/1 -> Terminator23/1
  Demux7/9 -> Terminator20/1
  Enabled Subsystem18/1(Out1) -> Goto67/1  "rawAzChecked"
  From89/1 -> Enabled Subsystem16/Enable
  Cos25/1 -> Product7/1
  Demux8/25 -> binary2double15/1(In1)
  Fletcher16 Checksum2/2(Out2) -> MATLAB Function8/4(cSumCalcB2)  "cSumCalcB2"
  binary2double10/1(Double) -> Enabled Subsystem10/1(Double), Goto70/1  "rawRoll"
  Selector1/1 -> Demux7/1
  Demux5/8 -> Fletcher16 Checksum/4(In4)
  [phiIMU] -> Cos25/1
  Demux/4 -> Display/1
  Constant/1 -> Sample and Hold2/Trigger, Integrator2/2, Sample and Hold/Trigger, Sample and Hold1/Trigger
  Demux8/39 -> binary2double18/3(In3)
  Demux8/21 -> binary2double14/1(In1)
  Divide/1 -> Sample and Hold2/1
  Demux/33 -> binary2double7/1(In1)
  Cos18/1 -> Product12/2
  Demux6/7 -> binary2double9/3(In3)
  Product12/1 -> Add5/1
  Demux/9 -> binary2double1/1(In1)
  Demux6/6 -> binary2double9/2(In2)
  Demux/17 -> binary2double3/1(In1)
  Demux4/1 -> Terminator8/1  "kiteP"
  Demux5/18 -> Fletcher16 Checksum/14(In14)
  Cos24/1 -> Product11/2
  binary2double15/1(Double) -> Enabled Subsystem15/1(Double), Goto53/1  "rawR"
  Product10/1 -> Add4/2
  [DcM] -> Matrix Multiply4/1
  Cos22/1 -> Product10/3
  Demux8/3 -> Display12/1
  Enabled Subsystem6/1(Out1) -> [axIMU]  "rawAxChecked"
  Demux/2 -> Display3/1
  Clock1/1 -> Sample and Hold1/1
  Demux5/3 -> Terminator13/1
  Demux5/7 -> Fletcher16 Checksum/3(In3)
  binary2double18/1(Double) -> Enabled Subsystem18/1(Double), Goto56/1  "rawAz"
  Demux8/44 -> binary2double19/4(In4)
  Demux9/22 -> Fletcher16 Checksum2/18(In18)
  Demux9/26 -> Fletcher16 Checksum2/22(In22)
  binary2double11/1(Double) -> Enabled Subsystem11/1(Double), Goto49/1  "rawPitch"
  Demux5/32 -> Fletcher16 Checksum/28(In28)
  Demux9/3 -> Terminator25/1
  Demux5/28 -> Fletcher16 Checksum/24(In24)
  Demux/20 -> binary2double3/4(In4)
  Demux5/2 -> Terminator12/1
  Gain13/1 -> Terminator33/1  "q"
  Ground/1 -> Fletcher16 Checksum/37(In37), Fletcher16 Checksum/38(In38), Fletcher16 Checksum/39(In39), Fletcher16 Checksum/40(In40)
  Demux/14 -> binary2double2/2(In2)
  [checksumEnable] -> Enabled Subsystem7/Enable
  Enabled Subsystem14/1(Out1) -> Goto62/1  "rawQchecked"
  From90/1 -> Enabled Subsystem17/Enable
  Cos20/1 -> Product8/2
  Demux6/3 -> Display6/1
  Mux1/1 -> Scope 2/1, eul/1
  Demux/43 -> Display1/1
  [psiIMU] -> Sum4/2
  Demux5/42 -> Terminator17/1
  Demux7/5 -> Fletcher16 Checksum1/1(In1)
  Demux9/28 -> Fletcher16 Checksum2/24(In24)
  Demux8/13 -> binary2double12/1(In1)
  Demux/13 -> binary2double2/1(In1)
  Gain1/1 -> Trigonometric Function4/1
  From72/1 -> Enabled Subsystem14/Enable
  Demux9/7 -> Fletcher16 Checksum2/3(In3)
  [checksumEnable] -> Enabled Subsystem/Enable
  Sum5/1 -> Cos15/1
  Demux4/2 -> [kiteQ], Terminator9/1  "kiteQ"
  Demux9/19 -> Fletcher16 Checksum2/15(In15)
  Cos14/1 -> Trigonometric Function3/1
  Demux8/20 -> binary2double13/4(In4)
  Fletcher16 Checksum1/1(Out1) -> MATLAB Function7/3(cSumCalcB1)  "cSumCalcB1"
  [kiteQ] -> Gain36/1
  Cos21/1 -> Product9/1
  Gain27/1 -> Mux4/3, Manual Switch1/1, Mux2/3  "yaw"
  Sin1/1 -> Product10/1
  [phiRaw] -> Gain11/1
  [psiIMU] -> Sum6/2
  From60/1 -> Enabled Subsystem13/Enable
  Gain25/1 -> Mux1/1, Mux2/1, Mux4/1  "roll"
  Demux9/41 -> Fletcher16 Checksum2/37(In37)
  Mux10/1 -> Reshape6/1
  Gain4/1 -> Add3/1  "rollRaw"
  Demux8/10 -> binary2double11/2(In2)
  Demux/24 -> binary2double4/4(In4)
  Enabled Subsystem3/1(Out1) -> [pIMU]  "rawPchecked"
  Enabled Subsystem4/1(Out1) -> [qIMU]  "rawQchecked"
  yawEstimateTrigger1/1 -> Integrator1/2
  Demux9/17 -> Fletcher16 Checksum2/13(In13)
  Demux/8 -> binary2double/4(In4)
  Demux8/32 -> binary2double16/4(In4)
  Add5/1 -> Trigonometric Function5/1
  PoolToNorthAngle1/1 -> Gain20/1
  Enabled Subsystem16/1(Out1) -> Goto64/1  "rawAxChecked"
  Demux8/1 -> Display14/1
  Ground1/1 -> Bus Creator2/3  "Pressure (Pa)"
  Demux/18 -> binary2double3/2(In2)
  Demux6/8 -> binary2double9/4(In4)
  binary2double12/1(Double) -> Enabled Subsystem12/1(Double), Goto50/1  "rawYaw"
  Sum6/1 -> Cos18/1
  Demux7/10 -> Terminator21/1
  Demux5/11 -> Fletcher16 Checksum/7(In7)
  Demux8/14 -> binary2double12/2(In2)
  [rateVector] -> angVel/1, Demux4/1
  Cos16/1 -> Product9/2
  Demux9/5 -> Fletcher16 Checksum2/1(In1)
  Demux9/10 -> Fletcher16 Checksum2/6(In6)
  "FIFO bin read "/1 -> Demux9/1, Demux8/1, Demux5/1, Demux/1
  Enabled Subsystem/1(Out1) -> [phiIMU]  "rawRollChecked"
  Selector/1 -> Demux6/1
  Demux9/40 -> Fletcher16 Checksum2/36(In36)
  Demux9/14 -> Fletcher16 Checksum2/10(In10)
  Demux9/16 -> Fletcher16 Checksum2/12(In12)
  Integrator2/1 -> Divide/1
  Sample and Hold/1 -> Sum/1
  Demux9/25 -> Fletcher16 Checksum2/21(In21)
  Demux/22 -> binary2double4/2(In2)
  [thetaIMU] -> Cos21/1
  From45/1 -> Enabled Subsystem11/Enable
  Demux9/33 -> Fletcher16 Checksum2/29(In29)
  Gain30/1 -> Mux3/4  "ax"
  Demux6/5 -> binary2double9/1(In1)
  binary2double6/1(Double) -> Enabled Subsystem6/1(Double), [axRaw]  "rawAx"
  MATLAB Function7/1(checksumIsMatching) -> Gain3/1
  Demux9/8 -> Fletcher16 Checksum2/4(In4)
  Demux8/47 -> Display11/1
  Demux5/31 -> Fletcher16 Checksum/27(In27)
  Demux8/28 -> binary2double15/4(In4)
  [thetaRaw] -> Gain32/1
  Demux5/41 -> Terminator16/1
  Demux5/17 -> Fletcher16 Checksum/13(In13)
  [CSisMatch] -> Terminator28/1  "CSisMatch"
  Enabled Subsystem5/1(Out1) -> [rIMU]  "rawRchecked"
  Demux5/34 -> Fletcher16 Checksum/30(In30)
  Demux9/47 -> Terminator32/1
  Demux8/22 -> binary2double14/2(In2)
  MATLAB Function8/1(checksumIsMatching) -> Gain31/1
  Demux9/45 -> Terminator30/1
  Demux7/6 -> Fletcher16 Checksum1/2(In2)
  Demux5/37 -> Fletcher16 Checksum/33(In33)
  eulRates/1 -> [rateVector], Bus Creator2/2  "gyroRates"
  Demux7/8 -> Fletcher16 Checksum1/4(In4)
  [checksumEnable] -> Enabled Subsystem1/Enable
  DcM/1 -> [DcM]
  Demux5/21 -> Fletcher16 Checksum/17(In17)
  binary2double5/1(Double) -> Enabled Subsystem5/1(Double), [rRaw]  "rawR"
  Demux8/41 -> binary2double19/1(In1)
  Fletcher16 Checksum2/1(Out1) -> MATLAB Function8/3(cSumCalcB1)  "cSumCalcB1"
  Demux/42 -> MATLAB Function6/2(cSumInB2)  "cSumInB2"
  Demux9/6 -> Fletcher16 Checksum2/2(In2)
  Gain18/1 -> Mux3/5  "ay"
  Gain3/1 -> [CSisMatchPressure], Cast To Boolean1/1  "checksumIsMatch"
  Demux7/3 -> Terminator10/1
  Demux9/4 -> Terminator26/1
  Reshape6/1 -> Matrix Multiply4/2
  Demux8/30 -> binary2double16/2(In2)
  Demux8/11 -> binary2double11/3(In3)
  Demux/10 -> binary2double1/2(In2)
  Saturation1/1 -> MATLAB Function3/2(theta)  "kitePitch_rad"
  Demux/6 -> binary2double/2(In2)
  Enabled Subsystem12/1(Out1) -> Goto59/1  "rawRollChecked"
  Demux6/11 -> Display9/1
  Enabled Subsystem8/1(Out1) -> [azIMU]  "rawAzChecked"
  yawBias1/1 -> Add3/2
  Demux5/26 -> Fletcher16 Checksum/22(In22)
  Demux/31 -> binary2double6/3(In3)
  Sum4/1 -> Cos22/1
  binary2double1/1(Double) -> Enabled Subsystem1/1(Double), [thetaRaw]  "rawPitch"
  [checksumEnable] -> Enabled Subsystem5/Enable
  MATLAB Function5/1(y) -> MATLAB Function3/3(q)
  Gain17/1 -> Mux3/7  "pressure"
  Demux9/43 -> Fletcher16 Checksum2/39(In39)
  Clock/1 -> Sample and Hold/1
  Demux8/18 -> binary2double13/2(In2)
  Demux8/15 -> binary2double12/3(In3)
  Demux9/46 -> Terminator31/1
  Enabled Subsystem17/1(Out1) -> Goto66/1  "rawAyChecked"
  Demux9/31 -> Fletcher16 Checksum2/27(In27)
  Demux9/38 -> Fletcher16 Checksum2/34(In34)
  Demux6/2 -> Display7/1
  From92/1 -> Enabled Subsystem19/Enable
  Demux/36 -> binary2double7/4(In4)
  Demux5/22 -> Fletcher16 Checksum/18(In18)
  Demux8/40 -> binary2double18/4(In4)
  Demux8/38 -> binary2double18/2(In2)
  binary2double19/1(Double) -> Enabled Subsystem19/1(Double)  "rawPressure"
  Demux9/30 -> Fletcher16 Checksum2/26(In26)
  Product11/1 -> Add4/1
  Demux5/30 -> Fletcher16 Checksum/26(In26)
  Demux9/29 -> Fletcher16 Checksum2/25(In25)
  [pres] -> Integrator2/1
  Demux/21 -> binary2double4/1(In1)
  Demux7/2 -> Terminator39/1
  Matrix Multiply4/1 -> Terminator37/1  "accBody"
  Demux9/34 -> Fletcher16 Checksum2/30(In30)
  Demux/19 -> binary2double3/3(In3)
  Demux5/19 -> Fletcher16 Checksum/15(In15)
  Cast To Boolean1/1 -> [checksumEnablePressure]
  [phiIMU] -> Cos24/1, Sin1/1
  serialData/1 -> "FIFO bin read "/1
  Bus Creator2/1 -> kiteMeasure/1  "kiteMeasure"

== system openWaterModel/Sensor Processing/Serial Unpacking/Subsystem ==
  In1 : Inport
  In2 : Inport  Port=2
  "Bit Packing " : xpcutilitieslib/Bit Packing   MaskBitPatterns={[0:15]}  MaskPackDataType=uint16  MaskPackDataSize=[1]
      settings: SourceProductBaseCode=XP
  Bit Packing 3 : xpcutilitieslib/Bit Packing   MaskBitPatterns={[0:7]}  MaskPackDataType=uint32  MaskPackDataSize=[1]
      settings: SourceProductBaseCode=XP
  Bit Packing 4 : xpcutilitieslib/Bit Packing   MaskBitPatterns={[0:7]}  MaskPackDataType=uint32  MaskPackDataSize=[1]
      settings: SourceProductBaseCode=XP
  Bit Shift3 : hdlsllib/Logic and Bit Operations/Bit Shift  mode=Shift Left Logical  N=8
  Bitwise Operator : simulink/Logic and Bit Operations/Bitwise Operator  logicop=OR  UseBitMask=off  NumInputPorts=2  BitMask=bin2dec('00000000')  BitMaskRealWorld=Stored Integer
  Cast To Double1 : DataTypeConversion  OutDataTypeStr=double
  Double : Outport
  wires:
  In1/1 -> Bit Packing 3/1
  Cast To Double1/1 -> Double/1
  Bit Packing 3/1 -> Bit Shift3/1
  Bit Packing 4/1 -> Bitwise Operator/2
  In2/1 -> Bit Packing 4/1
  Bitwise Operator/1 -> "Bit Packing "/1
  "Bit Packing "/1 -> Cast To Double1/1
  Bit Shift3/1 -> Bitwise Operator/1

== system openWaterModel/Sensor Processing/Serial Unpacking/Subsystem1 ==
  In1 : Inport
  In2 : Inport  Port=2
  "Bit Packing " : xpcutilitieslib/Bit Packing   MaskBitPatterns={[0:15]}  MaskPackDataType=uint16  MaskPackDataSize=[1]
      settings: SourceProductBaseCode=XP
  Bit Packing 3 : xpcutilitieslib/Bit Packing   MaskBitPatterns={[0:7]}  MaskPackDataType=uint32  MaskPackDataSize=[1]
      settings: SourceProductBaseCode=XP
  Bit Packing 4 : xpcutilitieslib/Bit Packing   MaskBitPatterns={[0:7]}  MaskPackDataType=uint32  MaskPackDataSize=[1]
      settings: SourceProductBaseCode=XP
  Bit Shift3 : hdlsllib/Logic and Bit Operations/Bit Shift  mode=Shift Left Logical  N=8
  Bitwise Operator : simulink/Logic and Bit Operations/Bitwise Operator  logicop=OR  UseBitMask=off  NumInputPorts=2  BitMask=bin2dec('00000000')  BitMaskRealWorld=Stored Integer
  Cast To Double1 : DataTypeConversion  OutDataTypeStr=double
  Double : Outport
  wires:
  In1/1 -> Bit Packing 3/1
  Cast To Double1/1 -> Double/1
  Bit Packing 3/1 -> Bit Shift3/1
  Bit Packing 4/1 -> Bitwise Operator/2
  In2/1 -> Bit Packing 4/1
  Bitwise Operator/1 -> "Bit Packing "/1
  "Bit Packing "/1 -> Cast To Double1/1
  Bit Shift3/1 -> Bitwise Operator/1

== system openWaterModel/Sensor Processing/Serial Unpacking/binary2double1 ==
  In3 : Inport
  In4 : Inport  Port=2
  "Bit Packing " : xpcutilitieslib/Bit Packing   Commented=through  MaskBitPatterns={[0:31]}  MaskPackDataType=single  MaskPackDataSize=[1]
      settings: SourceProductBaseCode=XP
  Bit Packing 3 : xpcutilitieslib/Bit Packing   MaskBitPatterns={[0:7]}  MaskPackDataType=uint16  MaskPackDataSize=[1]
      settings: SourceProductBaseCode=XP
  Bit Packing 4 : xpcutilitieslib/Bit Packing   MaskBitPatterns={[0:7]}  MaskPackDataType=uint16  MaskPackDataSize=[1]
      settings: SourceProductBaseCode=XP
  Bit Shift1 : hdlsllib/Logic and Bit Operations/Bit Shift  mode=Shift Left Logical  N=8
  Bitwise Operator : simulink/Logic and Bit Operations/Bitwise Operator  logicop=OR  UseBitMask=off  NumInputPorts=2  BitMask=bin2dec('00000000')  BitMaskRealWorld=Stored Integer
  Cast : DataTypeConversion  OutDataTypeStr=uint32
  Cast To Double1 : DataTypeConversion  OutDataTypeStr=double
  Display{1..4,6..7,12..13} (8 alike) : Display
      Display1 settings: Format=hex (Stored Integer)
      Display12 settings: Format=hex (Stored Integer)
      Display13 settings: Format=hex (Stored Integer)
      Display2 settings: Format=decimal (Stored Integer)
      Display3 settings: Format=decimal (Stored Integer)
      Display4 settings: Format=hex (Stored Integer)
      Display6 settings: Format=hex (Stored Integer)
      Display7 settings: Format=hex (Stored Integer)
  Double : Outport
  wires:
  Cast To Double1/1 -> Display3/1, Double/1
  In4/1 -> Display7/1, Bit Packing 4/1
  Bit Packing 3/1 -> Bitwise Operator/1, Display12/1
  In3/1 -> Display6/1, Bit Packing 3/1
  Bit Packing 4/1 -> Bit Shift1/1
  Bit Shift1/1 -> Bitwise Operator/2, Display13/1
  Bitwise Operator/1 -> Cast/1, Display1/1
  "Bit Packing "/1 -> Display2/1, Cast To Double1/1
  Cast/1 -> Display4/1, "Bit Packing "/1

== system openWaterModel/Sensor Processing/Serial Unpacking/binary2double2 ==
  In1 : Inport
  In2 : Inport  Port=2
  In3 : Inport  Port=3
  In4 : Inport  Port=4
  Bit Packing {1..5} (5 alike) : xpcutilitieslib/Bit Packing 
      settings: SourceProductBaseCode=XP
  Bit Shift1 : hdlsllib/Logic and Bit Operations/Bit Shift  mode=Shift Left Logical  N=16
  Bit Shift2 : hdlsllib/Logic and Bit Operations/Bit Shift  mode=Shift Left Logical  N=24
  Bit Shift3 : hdlsllib/Logic and Bit Operations/Bit Shift  mode=Shift Left Logical  N=8
  Bitwise Operator : simulink/Logic and Bit Operations/Bitwise Operator  logicop=OR  UseBitMask=off  NumInputPorts=4  BitMask=bin2dec('00000000')  BitMaskRealWorld=Stored Integer
  Cast To Double1 : DataTypeConversion  OutDataTypeStr=double
  Display{3,5..7,10..14} (9 alike) : Display
      settings: Format=hex (Stored Integer)
  Double : Outport
  wires:
  Cast To Double1/1 -> Double/1
  Bit Packing 3/1 -> Bit Shift3/1
  Bit Shift3/1 -> Display12/1, Bitwise Operator/3
  Bitwise Operator/1 -> Bit Packing 5/1, Display14/1
  Bit Packing 2/1 -> Bit Shift1/1
  Bit Shift2/1 -> Display11/1, Bitwise Operator/1
  Bit Packing 4/1 -> Display13/1, Bitwise Operator/4
  Bit Packing 1/1 -> Bit Shift2/1
  Bit Shift1/1 -> Display10/1, Bitwise Operator/2
  Bit Packing 5/1 -> Cast To Double1/1
  In1/1 -> Bit Packing 4/1, Display7/1
  In2/1 -> Bit Packing 3/1, Display6/1
  In3/1 -> Display5/1, Bit Packing 2/1
  In4/1 -> Bit Packing 1/1, Display3/1

== system openWaterModel/Sensor Processing/Serial Unpacking/binary2double5 ==
  In1 : Inport
  In2 : Inport  Port=2
  In3 : Inport  Port=3
  In4 : Inport  Port=4
  Bit Packing {,1..4} (5 alike) : xpcutilitieslib/Bit Packing 
      settings: SourceProductBaseCode=XP
  Bit Shift1 : hdlsllib/Logic and Bit Operations/Bit Shift  mode=Shift Left Logical  N=16
  Bit Shift2 : hdlsllib/Logic and Bit Operations/Bit Shift  mode=Shift Left Logical  N=24
  Bit Shift3 : hdlsllib/Logic and Bit Operations/Bit Shift  mode=Shift Left Logical  N=8
  Bitwise Operator : simulink/Logic and Bit Operations/Bitwise Operator  logicop=OR  UseBitMask=off  NumInputPorts=4  BitMask=bin2dec('00000000')  BitMaskRealWorld=Stored Integer
  Cast To Double1 : DataTypeConversion  OutDataTypeStr=double
  Display{3,5..7,10..14} (9 alike) : Display
      settings: Format=hex (Stored Integer)
  Double : Outport
  wires:
  Bit Shift1/1 -> Bitwise Operator/2, Display10/1
  Bitwise Operator/1 -> Display14/1, "Bit Packing "/1
  Bit Packing 1/1 -> Bit Shift2/1
  Bit Packing 4/1 -> Bitwise Operator/4, Display13/1
  In1/1 -> Bit Packing 1/1, Display3/1
  In3/1 -> Bit Packing 3/1, Display6/1
  Bit Shift2/1 -> Bitwise Operator/1, Display11/1
  Bit Packing 2/1 -> Bit Shift1/1
  "Bit Packing "/1 -> Cast To Double1/1
  Bit Shift3/1 -> Bitwise Operator/3, Display12/1
  Bit Packing 3/1 -> Bit Shift3/1
  In2/1 -> Bit Packing 2/1, Display5/1
  In4/1 -> Bit Packing 4/1, Display7/1
  Cast To Double1/1 -> Double/1

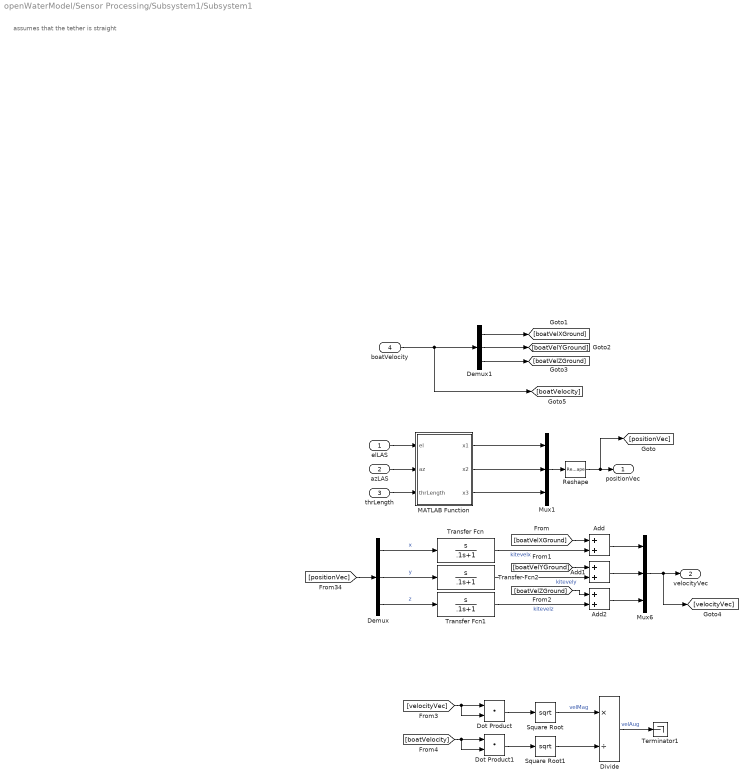
== system openWaterModel/Sensor Processing/Subsystem1/Subsystem1 ==
  note: assumes that the tether is straight
  elLAS : Inport
  azLAS : Inport  Port=2
  thrLength : Inport  Port=3
  boatVelocity : Inport  Port=4
  Add : Sum
  Add1 : Sum
  Add2 : Sum
  Demux : Demux  Outputs=3
  Demux1 : Demux  Outputs=3
  Divide : Product  Inputs=*/
  Dot Product : DotProduct  InputSameDT=on  OutDataTypeStr=Inherit: Inherit via internal rule
  Dot Product1 : DotProduct  InputSameDT=on  OutDataTypeStr=Inherit: Inherit via internal rule
  MATLAB Function : MATLAB Function  TreatAsAtomicUnit=on
  Mux1 : Mux  Inputs=3
  Mux6 : Mux  Inputs=3
  Reshape : Reshape  OutputDimensionality=Column vector (2-D)
  Square Root : Sqrt  SaturateOnIntegerOverflow=on
  Square Root1 : Sqrt  SaturateOnIntegerOverflow=on
  Terminator1 : Terminator
  Transfer Fcn : TransferFcn  Numerator=[1 0]  Denominator=[.1 1]
  Transfer Fcn1 : TransferFcn  Numerator=[1 0]  Denominator=[.1 1]
  Transfer Fcn2 : TransferFcn  Numerator=[1 0]  Denominator=[.1 1]
  positionVec : Outport
  velocityVec : Outport  Port=2
  wires:
  Reshape/1 -> [positionVec], positionVec/1
  [positionVec] -> Demux/1
  Mux6/1 -> [velocityVec], velocityVec/1
  Transfer Fcn/1 -> Add/2  "kitevelx"
  Transfer Fcn2/1 -> Add1/2  "kitevely"
  azLAS/1 -> MATLAB Function/2(az)
  MATLAB Function/2(x2) -> Mux1/2
  MATLAB Function/1(x1) -> Mux1/1
  thrLength/1 -> MATLAB Function/3(thrLength)
  elLAS/1 -> MATLAB Function/1(el)
  Mux1/1 -> Reshape/1
  Transfer Fcn1/1 -> Add2/2  "kitevelz"
  Demux/1 -> Transfer Fcn/1  "x"
  Demux/2 -> Transfer Fcn2/1  "y"
  Demux/3 -> Transfer Fcn1/1  "z"
  MATLAB Function/3(x3) -> Mux1/3
  Demux1/1 -> [boatVelXGround]
  Demux1/2 -> [boatVelYGround]
  Demux1/3 -> [boatVelZGround]
  [boatVelXGround] -> Add/1
  Add/1 -> Mux6/1
  [boatVelYGround] -> Add1/1
  Add1/1 -> Mux6/2
  [boatVelZGround] -> Add2/1
  Add2/1 -> Mux6/3
  [velocityVec] -> Dot Product/2, Dot Product/1
  Dot Product/1 -> Square Root/1
  Square Root/1 -> Divide/1  "velMag"
  Divide/1 -> Terminator1/1  "velAug"
  boatVelocity/1 -> [boatVelocity], Demux1/1
  Square Root1/1 -> Divide/2
  [boatVelocity] -> Dot Product1/1, Dot Product1/2
  Dot Product1/1 -> Square Root1/1

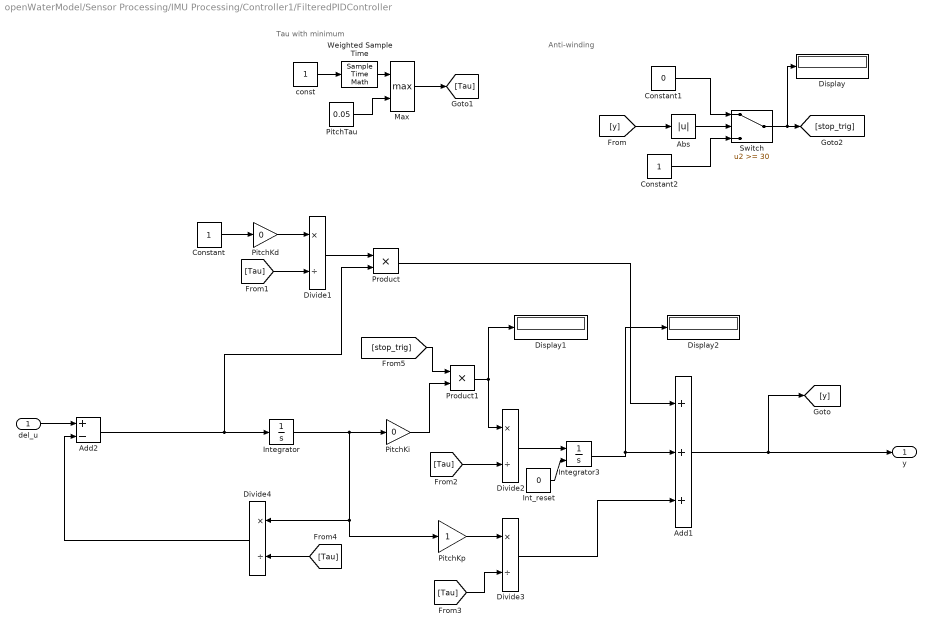
== system openWaterModel/Sensor Processing/IMU Processing/Controller1/FilteredPIDController ==
  note: Anti-winding
  note: Tau with minimum
  del_u : Inport
  Abs : Abs
  Add1 : Sum  Inputs=+++
  Add2 : Sum  Inputs=+-
  Constant : Constant
  Constant1 : Constant  Value=0
  Constant2 : Constant
  Display : Display
  Display1 : Display
  Display2 : Display
  Divide{1..4} (4 alike) : Product  Inputs=*/
  Int_reset : Constant  Value=0
  Integrator : Integrator
  Integrator3 : Integrator  ExternalReset=either
  Max : MinMax  Function=max  Inputs=2
  PitchKd : Gain  Gain=0
  PitchKi : Gain  Gain=0
  PitchKp : Gain
  PitchTau : Constant  Value=0.05
  Product : Product
  Product1 : Product
  Switch : Switch  Threshold=30
  Weighted Sample Time : SampleTimeMath  TsampMathOp=Ts Only
  const : Constant
  y : Outport
  wires:
  PitchTau/1 -> Max/2
  Add1/1 -> [y], y/1
  const/1 -> Weighted Sample Time/1
  Weighted Sample Time/1 -> Max/1
  Max/1 -> [Tau]
  PitchKd/1 -> Divide1/1
  Constant/1 -> PitchKd/1
  [Tau] -> Divide1/2
  Divide1/1 -> Product/1
  Integrator/1 -> PitchKp/1, Divide4/1, PitchKi/1
  [Tau] -> Divide2/2
  Divide2/1 -> Integrator3/1
  Integrator3/1 -> Display2/1, Add1/2
  Product/1 -> Add1/1
  PitchKp/1 -> Divide3/1
  Divide3/1 -> Add1/3
  [Tau] -> Divide3/2
  [Tau] -> Divide4/2
  del_u/1 -> Add2/1
  Divide4/1 -> Add2/2
  Add2/1 -> Product/2, Integrator/1
  [y] -> Abs/1
  Abs/1 -> Switch/2
  Constant1/1 -> Switch/1
  Constant2/1 -> Switch/3
  Switch/1 -> Display/1, [stop_trig]
  PitchKi/1 -> Product1/2
  [stop_trig] -> Product1/1
  Product1/1 -> Divide2/1, Display1/1
  Int_reset/1 -> Integrator3/2

== system openWaterModel/Sensor Processing/IMU Processing/Controller1/FilteredPIDController1 ==
  note: Anti-winding
  note: Tau with minimum
  del_u : Inport
  Abs : Abs
  Add1 : Sum  Inputs=+++
  Add2 : Sum  Inputs=+-
  Constant : Constant
  Constant1 : Constant  Value=0
  Constant2 : Constant
  Divide{1..4} (4 alike) : Product  Inputs=*/
  Int_reset : Constant  Value=0
  Integrator : Integrator
  Integrator3 : Integrator  ExternalReset=either
  Max : MinMax  Function=max  Inputs=2
  Product : Product
  Product1 : Product
  Switch : Switch  Threshold=30
  Weighted Sample Time : SampleTimeMath  TsampMathOp=Ts Only
  YawKd : Gain  Gain=0.05
  YawKi : Gain  Gain=0
  YawKp : Gain  Gain=0.3
  YawTau : Constant  Value=0.02
  const : Constant
  y : Outport
  wires:
  YawTau/1 -> Max/2
  Add1/1 -> [y], y/1
  const/1 -> Weighted Sample Time/1
  Weighted Sample Time/1 -> Max/1
  Max/1 -> [Tau]
  YawKd/1 -> Divide1/1
  Constant/1 -> YawKd/1
  [Tau] -> Divide1/2
  Divide1/1 -> Product/1
  Integrator/1 -> YawKp/1, Divide4/1, YawKi/1
  [Tau] -> Divide2/2
  Divide2/1 -> Integrator3/1
  Integrator3/1 -> Add1/2
  Product/1 -> Add1/1
  YawKp/1 -> Divide3/1
  Divide3/1 -> Add1/3
  [Tau] -> Divide3/2
  [Tau] -> Divide4/2
  del_u/1 -> Add2/1
  Divide4/1 -> Add2/2
  Add2/1 -> Product/2, Integrator/1
  [y] -> Abs/1
  Abs/1 -> Switch/2
  Constant1/1 -> Switch/1
  Constant2/1 -> Switch/3
  Switch/1 -> [stop_trig]
  YawKi/1 -> Product1/2
  [stop_trig] -> Product1/1
  Product1/1 -> Divide2/1
  Int_reset/1 -> Integrator3/2
